simulink model "Adaptive_MPCbad"  (R2018b)
settings: Solver=FixedStepAuto  StartTime=0.0  StopTime=480  FixedStep=0.1  RelTol=1e-3
libraries: simulink x2, mpclib x1
settings Model: Creator=mulusoy  LastModifiedBy=Lenovo X250
settings OptimizationCC: DefaultParameterBehavior=Inlined  EnhancedBackFolding=on  PassReuseOutputArgsAs=Individual arguments  OptimizeBlockOrder=speed  DifferentSizesBufferReuse=on  OptimizationCustomize=off
settings DebuggingCC: ParameterTunabilityLossMsg=error  LibraryContextMissingDiagnostic=none
settings SFSimCC: SimUseLocalCustomCode=off  MATLABDynamicMemAlloc=off
settings RTWCC: SystemTargetFile=ert.tlc  TemplateMakefile=ert_default_tmf  GenerateReport=on  RTWUseLocalCustomCode=off  IncludeHyperlinkInReport=on  LaunchReport=on  GenerateTraceInfo=on  GenerateTraceReport=on  GenerateTraceReportSl=on  GenerateTraceReportSf=on  GenerateTraceReportEml=on
settings CodeAppCC: ForceParamTrailComments=on  IgnoreCustomStorageClasses=off  OperatorAnnotations=on  SimulinkDataObjDesc=on  SFDataObjDesc=on  InsertBlockDesc=on
settings ERTTargetCC: TargetLangStandard=C99 (ISO)  GenerateSampleERTMain=on  InlinedParameterPlacement=NonHierarchical  ERTCustomFileTemplate=example_file_process.tlc

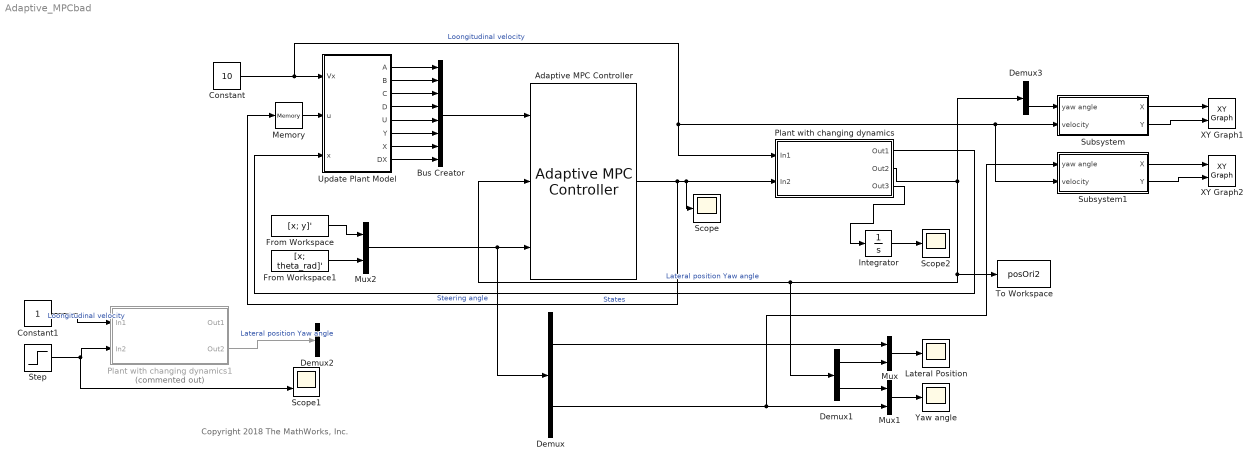
== system Adaptive_MPCbad ==
  note: Copyright 2018 The MathWorks, Inc.
  Adaptive MPC Controller : mpclib/Adaptive MPC Controller  SCDEnableBlockLinearizationSpecification=on  mpcobj=mpc1  enable_value=0  updateMPCinCallerWorkspace=on  md_inport=off  mv_inport=off  return_cost=off  return_mvseq=off  return_qpstatus=off  return_xseq=off  return_state=off  return_ovseq=off  state_inport=off  isltv_plant=off  umin_inport=off  umax_inport=off  ymin_inport=off  ymax_inport=off  cc_inport=off  ywt_inport=off  uwt_inport=off  duwt_inport=off  rhoeps_inport=off  uref_inport=off  BlockDataType=double  SampleTimeInherited=off  switch_inport=off
      settings: SourceProductName=Model Predictive Control Toolbox
  Bus Creator : BusCreator  Inputs=8
  Constant : Constant  Value=10
  Constant1 : Constant
  Demux{,1..3} (4 alike) : Demux  Outputs=2
  From Workspace : FromWorkspace  VariableName=[x; y]'  OutDataTypeStr=double  SampleTime=0
  From Workspace1 : FromWorkspace  VariableName=[x; theta_rad]'  OutDataTypeStr=double  SampleTime=0
  Integrator : Integrator
  Lateral Position : Scope
  Memory : Memory
  Mux : Mux  Inputs=2
  Mux1 : Mux  Inputs=2
  Mux2 : Mux  Inputs=2
  Plant with changing dynamics : Subsystem
      mask Display: image('car.jpg');
  Plant with changing dynamics1 : Subsystem  Commented=on
      mask Display: image('car.jpg');
  Scope : Scope
  Scope1 : Scope  NumInputPorts=2
  Scope2 : Scope
  Step : Step  SampleTime=0
  Subsystem : Subsystem
  Subsystem1 : Subsystem
  To Workspace : ToWorkspace  VariableName=posOri2  SampleTime=-1
  Update Plant Model : MATLAB Function  TreatAsAtomicUnit=on
  XY Graph1 : simulink/Sinks/XY Graph  xmin=-500  xmax=500  ymin=-500  ymax=500  st=-1
  XY Graph2 : simulink/Sinks/XY Graph  xmin=-500  xmax=500  ymin=-500  ymax=500  st=-1
  Yaw angle : Scope
  wires:
  Constant/1 -> Subsystem1/2(velocity), Subsystem/2(velocity), Plant with changing dynamics/1(In1), Update Plant Model/1(Vx)  "Loongitudinal velocity"
  Update Plant Model/1(A) -> Bus Creator/1
  Update Plant Model/2(B) -> Bus Creator/2
  Update Plant Model/3(C) -> Bus Creator/3
  Update Plant Model/4(D) -> Bus Creator/4
  Update Plant Model/5(U) -> Bus Creator/5
  Update Plant Model/6(Y) -> Bus Creator/6
  Update Plant Model/7(X) -> Bus Creator/7
  Update Plant Model/8(DX) -> Bus Creator/8
  Bus Creator/1 -> Adaptive MPC Controller/1
  Adaptive MPC Controller/1 -> Memory/1, Scope/1, Plant with changing dynamics/2(In2)  "Steering angle"
  Demux/1 -> Mux/1
  Mux/1 -> Lateral Position/1
  Demux1/1 -> Mux/2
  Demux1/2 -> Mux1/1
  Demux/2 -> Subsystem1/1(yaw angle), Mux1/2
  Mux1/1 -> Yaw angle/1
  Plant with changing dynamics/1(Out1) -> Update Plant Model/3(x)  "States"
  Memory/1 -> Update Plant Model/2(u)
  From Workspace/1 -> Mux2/1
  From Workspace1/1 -> Mux2/2
  Mux2/1 -> Demux/1, Adaptive MPC Controller/3
  Step/1 -> Scope1/2, Plant with changing dynamics1/2(In2)
  Constant1/1 -> Plant with changing dynamics1/1(In1)  "Loongitudinal velocity"
  Plant with changing dynamics1/2(Out2) -> Demux2/1  "Lateral position Yaw angle"
  Plant with changing dynamics/2(Out2) -> To Workspace/1, Demux1/1, Adaptive MPC Controller/2, Demux3/1  "Lateral position Yaw angle"
  Demux3/2 -> Subsystem/1(yaw angle)
  Subsystem/1(X) -> XY Graph1/1
  Subsystem/2(Y) -> XY Graph1/2
  Subsystem1/1(X) -> XY Graph2/1
  Subsystem1/2(Y) -> XY Graph2/2
  Plant with changing dynamics/3(Out3) -> Integrator/1
  Integrator/1 -> Scope2/1

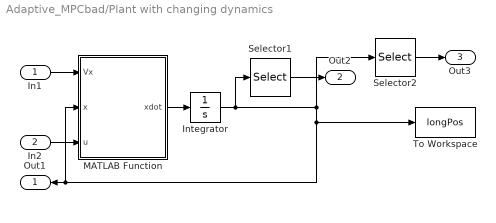
== system Adaptive_MPCbad/Plant with changing dynamics ==
  In1 : Inport
  In2 : Inport  Port=2
  Integrator : Integrator
  MATLAB Function : MATLAB Function  TreatAsAtomicUnit=on
  Selector1 : Selector  InputPortWidth=4  IndexOptions=Index vector (dialog)  Indices=[4 2]  OutputSizes=1
  Selector2 : Selector  InputPortWidth=4  IndexOptions=Index vector (dialog)  Indices=[3]  OutputSizes=1
  To Workspace : ToWorkspace  VariableName=longPos  SaveFormat=Timeseries  SampleTime=-1
  Out1 : Outport
  Out2 : Outport  Port=2
  Out3 : Outport  Port=3
  wires:
  In2/1 -> MATLAB Function/3(u)
  In1/1 -> MATLAB Function/1(Vx)
  MATLAB Function/1(xdot) -> Integrator/1
  Selector1/1 -> Out2/1
  Integrator/1 -> Selector1/1, To Workspace/1, MATLAB Function/2(x), Out1/1, Selector2/1
  Selector2/1 -> Out3/1

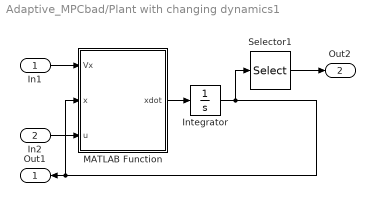
== system Adaptive_MPCbad/Plant with changing dynamics1 ==
  In1 : Inport
  In2 : Inport  Port=2
  Integrator : Integrator
  MATLAB Function : MATLAB Function  TreatAsAtomicUnit=on
  Selector1 : Selector  InputPortWidth=4  IndexOptions=Index vector (dialog)  Indices=[4 2]  OutputSizes=1
  Out1 : Outport
  Out2 : Outport  Port=2
  wires:
  In2/1 -> MATLAB Function/3(u)
  In1/1 -> MATLAB Function/1(Vx)
  MATLAB Function/1(xdot) -> Integrator/1
  Selector1/1 -> Out2/1
  Integrator/1 -> Selector1/1, MATLAB Function/2(x), Out1/1

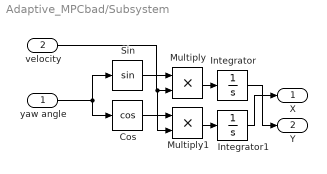
== system Adaptive_MPCbad/Subsystem ==
  yaw angle : Inport
  velocity : Inport  Port=2
  Cos : Trigonometry  Operator=cos
  Integrator : Integrator
  Integrator1 : Integrator
  Multiply : Product
  Multiply1 : Product
  Sin : Trigonometry
  X : Outport
  Y : Outport  Port=2
  wires:
  Multiply1/1 -> Integrator1/1
  Cos/1 -> Multiply1/1
  Sin/1 -> Multiply/1
  Multiply/1 -> Integrator/1
  Integrator1/1 -> X/1
  Integrator/1 -> Y/1
  yaw angle/1 -> Sin/1, Cos/1
  velocity/1 -> Multiply1/2, Multiply/2

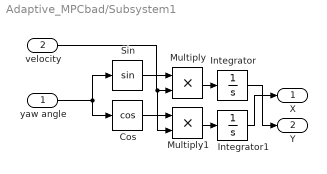
== system Adaptive_MPCbad/Subsystem1 ==
  yaw angle : Inport
  velocity : Inport  Port=2
  Cos : Trigonometry  Operator=cos
  Integrator : Integrator
  Integrator1 : Integrator
  Multiply : Product
  Multiply1 : Product
  Sin : Trigonometry
  X : Outport
  Y : Outport  Port=2
  wires:
  Multiply1/1 -> Integrator1/1
  Cos/1 -> Multiply1/1
  Sin/1 -> Multiply/1
  Multiply/1 -> Integrator/1
  Integrator1/1 -> X/1
  Integrator/1 -> Y/1
  yaw angle/1 -> Sin/1, Cos/1
  velocity/1 -> Multiply1/2, Multiply/2

== matlab function Adaptive_MPCbad/Plant with changing dynamics/MATLAB Function ==
  data: Vx input; x input size=[4,1]; u input; xdot output size=[4,1]
function xdot = fcn(Vx,x,u)

% Model parameters
m = 1575;
Iz = 2875;
lf = 1.2;
lr = 1.6;
Cf = 19000;
Cr = 33000;

% Continuous-time model
A = [-(2*Cf+2*Cr)/m/Vx, 0, -Vx-(2*Cf*lf-2*Cr*lr)/m/Vx, 0;
     0, 0, 1, 0;
     -(2*Cf*lf-2*Cr*lr)/Iz/Vx, 0, -(2*Cf*lf^2+2*Cr*lr^2)/Iz/Vx, 0;
     1, Vx, 0, 0];
B = [2*Cf/m 0 2*Cf*lf/Iz 0]';  
C = [0 0 0 1; 0 1 0 0];
D = zeros(2,1);
xdot = A*x + B*u;
%y = C*x + D*u;

== matlab function Adaptive_MPCbad/Update Plant Model ==
  data: Vx input; u input; A output size=[4,4]; x input size=[4,1]; B output size=[4,1]; C output size=[2,4]; D output size=[2,1]; U output; Y output size=[2,1]; X output size=[4,1]; DX output size=[4,1]
function [A,B,C,D,U,Y,X,DX] = fcn(Vx,u,x)
% Sample time
Ts = 0.1;

% Model parameters
m = 1575;
Iz = 2875;
lf = 1.2;
lr = 1.6;
Cf = 19000;
Cr = 33000;

% Continuous-time model
Ac = [-(2*Cf+2*Cr)/m/Vx, 0, -Vx-(2*Cf*lf-2*Cr*lr)/m/Vx, 0;
     0, 0, 1, 0;
     -(2*Cf*lf-2*Cr*lr)/Iz/Vx, 0, -(2*Cf*lf^2+2*Cr*lr^2)/Iz/Vx, 0;
     1, Vx, 0, 0];
Bc = [2*Cf/m 0 2*Cf*lf/Iz 0]';   
Cc = [0 0 0 1; 0 1 0 0];
Dc = zeros(2,1);

% Generate discrete-time model
nx = size(Ac,1);
nu = size(Bc,2);
M = expm([[Ac Bc]*Ts; zeros(nu,nx+nu)]);
A = M(1:nx,1:nx);
B = M(1:nx,nx+1:nx+nu);
C = Cc;
D = Dc;

% Nominal conditions for discrete-time plant
X = x;
U = u;
Y = C*x + D*u;
DX = A*x+B*u-x;

== matlab function Adaptive_MPCbad/Plant with changing dynamics1/MATLAB Function ==
  data: Vx input; x input size=[4,1]; u input; xdot output size=[4,1]
function xdot = fcn(Vx,x,u)

% Model parameters
m = 1575;
Iz = 2875;
lf = 1.2;
lr = 1.6;
Cf = 19000;
Cr = 33000;

% Continuous-time model
A = [-(2*Cf+2*Cr)/m/Vx, 0, -Vx-(2*Cf*lf-2*Cr*lr)/m/Vx, 0;
     0, 0, 1, 0;
     -(2*Cf*lf-2*Cr*lr)/Iz/Vx, 0, -(2*Cf*lf^2+2*Cr*lr^2)/Iz/Vx, 0;
     1, Vx, 0, 0];
B = [2*Cf/m 0 2*Cf*lf/Iz 0]';  
C = [0 0 0 1; 0 1 0 0];
D = zeros(2,1);
xdot = A*x + B*u;
%y = C*x + D*u;
